simulink model "mdl5"  (R2014a)
settings: Solver=FixedStepDiscrete  SolverMode=SingleTasking  StartTime=TIME(1)  StopTime=TIME(end)  FixedStep=SIMSTEP  RelTol=1e-3
model workspace (MAT data in the model file):
  autoc_mdd_data01 : struct (value not decoded)
values from neighbouring files (symbols this model uses):
  map_mr4_01 = [400 500 600 700 800 900 1000 1100 1200 1300 1400 1500 ... (47 elements, 1x47)]    [scr_simdata_all.mat]
  map_mr4_02 = [0.684 0.622 0.566 0.514 0.468 0.425 0.387 0.352 0.32 0.291 0.264 0.241 ... (47 elements, 1x47)]    [scr_simdata_all.mat]
  map_mr4_03 = [10 12 14 16 18 20 22 24 26 28 30 32 ... (51 elements, 1x51)]    [scr_simdata_all.mat]
  map_mr4_04 = [0.0257 0.0124 0.00595 0.00286 0.00137 0.000662 0.000318 0.000153 7.37e-05 3.54e-05 1.7e-05 8.19e-06 ... (51 elements, 1x51)]    [scr_simdata_all.mat]
  map_mr4_05 = [10 12 14 16 18 20 22 24 26 28 30 32 ... (51 elements, 1x51)]    [scr_simdata_all.mat]
  map_mr4_06 = [0.9647 0.9835 0.9945 0.9994 0.9972 0.9871 0.97 0.9462 0.9163 0.8807 0.8403 0.796 ... (51 elements, 1x51)]    [scr_simdata_all.mat]
  map_mr4_07 = [0 1 2 3 4 5 6 7 8 9 10 11 ... (51 elements, 1x51)]    [scr_simdata_all.mat]
  map_mr4_08 = [0 0.01 0.0214 0.0335 0.0459 0.0587 0.0718 0.085 0.0985 0.112 0.126 0.14 ... (51 elements, 1x51)]    [scr_simdata_all.mat]
  Parameter114 = 126    [scr_simdata_all.mat]
  Parameter115 = 129    [scr_simdata_all.mat]
  Parameter131 = 3    [scr_simdata_all.mat]
  Parameter141 = 0    [scr_simdata_all.mat]
  Parameter143 = 1    [scr_simdata_all.mat]
  Parameter144 = 3    [scr_simdata_all.mat]
  Parameter51 = 0    [scr_simdata_all.mat]
  Parameter52 = 1    [scr_simdata_all.mat]
  Parameter53 = 2    [scr_simdata_all.mat]
  Parameter70 = 30    [scr_simdata_all.mat]
  Parameter71 = 33    [scr_simdata_all.mat]
  Parameter92 = 78    [scr_simdata_all.mat]
  Parameter93 = 81    [scr_simdata_all.mat]
  SIMSTEP = 0.0001024    [scr_simdata_all.mat]
(part 3 of 4)

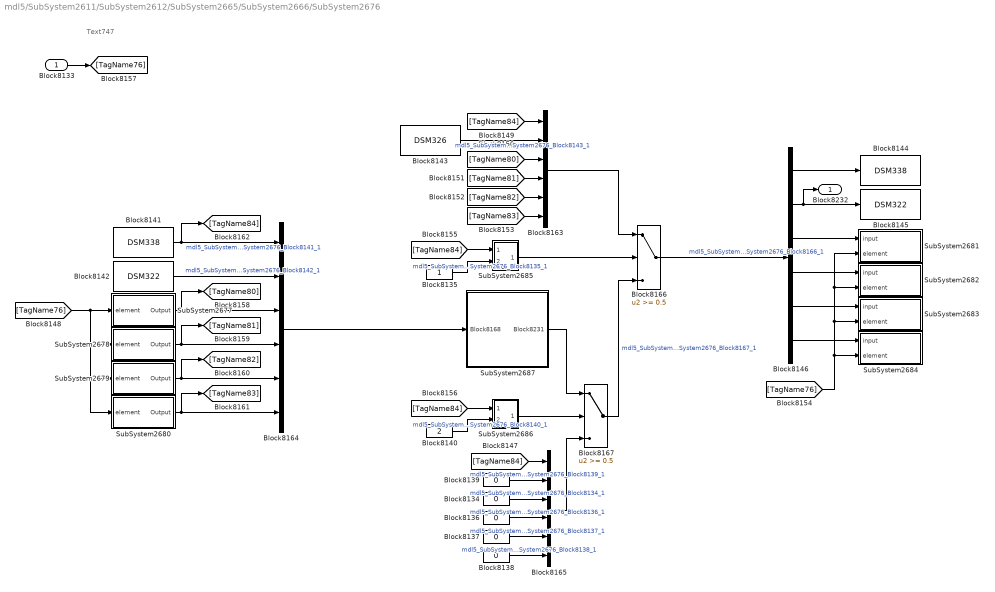
== system mdl5/SubSystem2611/SubSystem2612/SubSystem2665/SubSystem2666/SubSystem2676 ==
  note: Text747
  Block8133 : Inport
  Block{8134,8136..8139} (5 alike) : Constant  Value=0  OutDataTypeStr=double  SampleTime=-1
  Block8135 : Constant  OutDataTypeStr=double  SampleTime=-1
  Block8140 : Constant  Value=2  OutDataTypeStr=double  SampleTime=-1
  Block8141 : DataStoreRead  DataStoreName=DSM338
  Block8142 : DataStoreRead  DataStoreName=DSM322
  Block8143 : DataStoreRead  DataStoreName=DSM326
  Block8144 : DataStoreWrite  DataStoreName=DSM338
  Block8145 : DataStoreWrite  DataStoreName=DSM322
  Block8146 : Demux  Outputs=6
  Block8163 : Mux  Inputs=6
  Block8164 : Mux  Inputs=6
  Block8165 : Mux  Inputs=6
  Block8166 : Switch  Threshold=0.5  RndMeth=Zero  SaturateOnIntegerOverflow=on  InputSameDT=on
  Block8167 : Switch  Threshold=0.5  RndMeth=Zero  SaturateOnIntegerOverflow=on  InputSameDT=on
  SubSystem2677 : Subsystem  TreatAsAtomicUnit=on  mask(***ATC.DSRVEC***){bd_version=1.01.A, r0=DSM334, r1=-1, r2=, r3=, r4=, r5=, r6=, r7=, r8=, r9=, c0=, c1=, c2=, c3=, c4=, c5=, c6=, c7=, c8=, c9=}
      mask prompts: bd_version "Version"
      mask help: これはAutoCからのブロックです．編集禁止．
      settings: OpenFcn=warndlg('変更禁止!');
      mask Help: web(ui_blockhelpmng(gcb));
      mask Display: disp('ATC.DSRVEC')
  SubSystem2678 : Subsystem  TreatAsAtomicUnit=on  mask(***ATC.DSRVEC***){bd_version=1.01.A, r0=DSM335, r1=-1, r2=, r3=, r4=, r5=, r6=, r7=, r8=, r9=, c0=, c1=, c2=, c3=, c4=, c5=, c6=, c7=, c8=, c9=}
      mask prompts: bd_version "Version"
      mask help: これはAutoCからのブロックです．編集禁止．
      settings: OpenFcn=warndlg('変更禁止!');
      mask Help: web(ui_blockhelpmng(gcb));
      mask Display: disp('ATC.DSRVEC')
  SubSystem2679 : Subsystem  TreatAsAtomicUnit=on  mask(***ATC.DSRVEC***){bd_version=1.01.A, r0=DSM336, r1=-1, r2=, r3=, r4=, r5=, r6=, r7=, r8=, r9=, c0=, c1=, c2=, c3=, c4=, c5=, c6=, c7=, c8=, c9=}
      mask prompts: bd_version "Version"
      mask help: これはAutoCからのブロックです．編集禁止．
      settings: OpenFcn=warndlg('変更禁止!');
      mask Help: web(ui_blockhelpmng(gcb));
      mask Display: disp('ATC.DSRVEC')
  SubSystem2680 : Subsystem  TreatAsAtomicUnit=on  mask(***ATC.DSRVEC***){bd_version=1.01.A, r0=DSM337, r1=-1, r2=, r3=, r4=, r5=, r6=, r7=, r8=, r9=, c0=, c1=, c2=, c3=, c4=, c5=, c6=, c7=, c8=, c9=}
      mask prompts: bd_version "Version"
      mask help: これはAutoCからのブロックです．編集禁止．
      settings: OpenFcn=warndlg('変更禁止!');
      mask Help: web(ui_blockhelpmng(gcb));
      mask Display: disp('ATC.DSRVEC')
  SubSystem2681 : Subsystem  TreatAsAtomicUnit=on  mask(***ATC.DSWVEC***){bd_version=1.01.A, r0=DSM334, r1=-1, r2=, r3=, r4=, r5=, r6=, r7=, r8=, r9=, c0=, c1=, c2=, c3=, c4=, c5=, c6=, c7=, c8=, c9=}
      mask prompts: bd_version "Version"
      mask help: これはAutoCからのブロックです．編集禁止．
      settings: OpenFcn=warndlg('変更禁止!');
      mask Help: web(ui_blockhelpmng(gcb));
      mask Display: disp('ATC.DSRVEC')
  SubSystem2682 : Subsystem  TreatAsAtomicUnit=on  mask(***ATC.DSWVEC***){bd_version=1.01.A, r0=DSM335, r1=-1, r2=, r3=, r4=, r5=, r6=, r7=, r8=, r9=, c0=, c1=, c2=, c3=, c4=, c5=, c6=, c7=, c8=, c9=}
      mask prompts: bd_version "Version"
      mask help: これはAutoCからのブロックです．編集禁止．
      settings: OpenFcn=warndlg('変更禁止!');
      mask Help: web(ui_blockhelpmng(gcb));
      mask Display: disp('ATC.DSRVEC')
  SubSystem2683 : Subsystem  TreatAsAtomicUnit=on  mask(***ATC.DSWVEC***){bd_version=1.01.A, r0=DSM336, r1=-1, r2=, r3=, r4=, r5=, r6=, r7=, r8=, r9=, c0=, c1=, c2=, c3=, c4=, c5=, c6=, c7=, c8=, c9=}
      mask prompts: bd_version "Version"
      mask help: これはAutoCからのブロックです．編集禁止．
      settings: OpenFcn=warndlg('変更禁止!');
      mask Help: web(ui_blockhelpmng(gcb));
      mask Display: disp('ATC.DSRVEC')
  SubSystem2684 : Subsystem  TreatAsAtomicUnit=on  mask(***ATC.DSWVEC***){bd_version=1.01.A, r0=DSM337, r1=-1, r2=, r3=, r4=, r5=, r6=, r7=, r8=, r9=, c0=, c1=, c2=, c3=, c4=, c5=, c6=, c7=, c8=, c9=}
      mask prompts: bd_version "Version"
      mask help: これはAutoCからのブロックです．編集禁止．
      settings: OpenFcn=warndlg('変更禁止!');
      mask Help: web(ui_blockhelpmng(gcb));
      mask Display: disp('ATC.DSRVEC')
  SubSystem2685 : Subsystem
  SubSystem2686 : Subsystem
  SubSystem2687 : Subsystem  TreatAsAtomicUnit=on
  Block8232 : Outport
  wires:
  [TagName76] -> SubSystem2681/2(element), SubSystem2682/2(element), SubSystem2683/2(element), SubSystem2684/2(element)
  SubSystem2687/1(Block8231) -> Block8167/1
  Block8133/1 -> [TagName76]
  Block8164/1 -> SubSystem2687/1(Block8168)
  Block8141/1 -> [TagName84], Block8164/1  "mdl5_SubSystem2611_SubSystem2612_SubSystem2665_SubSystem2666_SubSystem2676_Block8141_1"
  Block8142/1 -> Block8164/2  "mdl5_SubSystem2611_SubSystem2612_SubSystem2665_SubSystem2666_SubSystem2676_Block8142_1"
  SubSystem2677/1(Output) -> [TagName80], Block8164/3
  SubSystem2678/1(Output) -> [TagName81], Block8164/4
  SubSystem2679/1(Output) -> [TagName82], Block8164/5
  SubSystem2680/1(Output) -> [TagName83], Block8164/6
  [TagName84] -> SubSystem2685/1(In1)
  Block8135/1 -> SubSystem2685/2(In2)  "mdl5_SubSystem2611_SubSystem2612_SubSystem2665_SubSystem2666_SubSystem2676_Block8135_1"
  [TagName84] -> SubSystem2686/1(In1)
  Block8140/1 -> SubSystem2686/2(In2)  "mdl5_SubSystem2611_SubSystem2612_SubSystem2665_SubSystem2666_SubSystem2676_Block8140_1"
  SubSystem2685/1(Out1) -> Block8166/2
  SubSystem2686/1(Out1) -> Block8167/2
  Block8163/1 -> Block8166/1
  Block8165/1 -> Block8167/3
  [TagName76] -> SubSystem2677/1(element), SubSystem2678/1(element), SubSystem2679/1(element), SubSystem2680/1(element)
  Block8166/1 -> Block8146/1  "mdl5_SubSystem2611_SubSystem2612_SubSystem2665_SubSystem2666_SubSystem2676_Block8166_1"
  Block8167/1 -> Block8166/3  "mdl5_SubSystem2611_SubSystem2612_SubSystem2665_SubSystem2666_SubSystem2676_Block8167_1"
  Block8146/1 -> Block8144/1
  Block8146/2 -> Block8145/1, Block8232/1
  Block8146/3 -> SubSystem2681/1(input)
  Block8146/4 -> SubSystem2682/1(input)
  Block8146/5 -> SubSystem2683/1(input)
  Block8146/6 -> SubSystem2684/1(input)
  [TagName84] -> Block8163/1
  Block8143/1 -> Block8163/2  "mdl5_SubSystem2611_SubSystem2612_SubSystem2665_SubSystem2666_SubSystem2676_Block8143_1"
  [TagName80] -> Block8163/3
  [TagName81] -> Block8163/4
  [TagName82] -> Block8163/5
  [TagName83] -> Block8163/6
  [TagName84] -> Block8165/1
  Block8139/1 -> Block8165/2  "mdl5_SubSystem2611_SubSystem2612_SubSystem2665_SubSystem2666_SubSystem2676_Block8139_1"
  Block8134/1 -> Block8165/3  "mdl5_SubSystem2611_SubSystem2612_SubSystem2665_SubSystem2666_SubSystem2676_Block8134_1"
  Block8136/1 -> Block8165/4  "mdl5_SubSystem2611_SubSystem2612_SubSystem2665_SubSystem2666_SubSystem2676_Block8136_1"
  Block8137/1 -> Block8165/5  "mdl5_SubSystem2611_SubSystem2612_SubSystem2665_SubSystem2666_SubSystem2676_Block8137_1"
  Block8138/1 -> Block8165/6  "mdl5_SubSystem2611_SubSystem2612_SubSystem2665_SubSystem2666_SubSystem2676_Block8138_1"

== system mdl5/SubSystem2611/SubSystem2691/SubSystem2693/SubSystem2695/SubSystem2696 ==
  note: ***編集禁止***
  input : Inport
  element : Inport  Port=2
  Assignment : Assignment  IndexOptions=Index vector (port)  OutputSizes=[1 1]
  Inside_DSR : DataStoreRead  DataStoreName=DSM320
  Inside_DSW : DataStoreWrite  DataStoreName=DSM320
  wires:
  Assignment/1 -> Inside_DSW/1  "mdl5_SubSystem2611_SubSystem2691_SubSystem2693_SubSystem2695_SubSystem2696_Assignment_1"
  Inside_DSR/1 -> Assignment/1  "mdl5_SubSystem2611_SubSystem2691_SubSystem2693_SubSystem2695_SubSystem2696_Inside_DSR_1"
  input/1 -> Assignment/2
  element/1 -> Assignment/3

== system mdl5/SubSystem2611/SubSystem2691/SubSystem2693/SubSystem2695/SubSystem2697 ==
  note: ***編集禁止***
  input : Inport
  element : Inport  Port=2
  Assignment : Assignment  IndexOptions=Index vector (port)  OutputSizes=[1 1]
  Inside_DSR : DataStoreRead  DataStoreName=DSM319
  Inside_DSW : DataStoreWrite  DataStoreName=DSM319
  wires:
  Assignment/1 -> Inside_DSW/1  "mdl5_SubSystem2611_SubSystem2691_SubSystem2693_SubSystem2695_SubSystem2697_Assignment_1"
  Inside_DSR/1 -> Assignment/1  "mdl5_SubSystem2611_SubSystem2691_SubSystem2693_SubSystem2695_SubSystem2697_Inside_DSR_1"
  input/1 -> Assignment/2
  element/1 -> Assignment/3

== system mdl5/SubSystem2611/SubSystem2691/SubSystem2693/SubSystem2695/SubSystem2698 ==
  note: ***編集禁止***
  input : Inport
  element : Inport  Port=2
  Assignment : Assignment  IndexOptions=Index vector (port)  OutputSizes=[1 1]
  Inside_DSR : DataStoreRead  DataStoreName=DSM336
  Inside_DSW : DataStoreWrite  DataStoreName=DSM336
  wires:
  element/1 -> Assignment/3
  input/1 -> Assignment/2
  Inside_DSR/1 -> Assignment/1  "mdl5_SubSystem2611_SubSystem2691_SubSystem2693_SubSystem2695_SubSystem2698_Inside_DSR_1"
  Assignment/1 -> Inside_DSW/1  "mdl5_SubSystem2611_SubSystem2691_SubSystem2693_SubSystem2695_SubSystem2698_Assignment_1"

== system mdl5/SubSystem2611/SubSystem2691/SubSystem2693/SubSystem2695/SubSystem2699 ==
  note: ***編集禁止***
  input : Inport
  element : Inport  Port=2
  Assignment : Assignment  IndexOptions=Index vector (port)  OutputSizes=[1 1]
  Inside_DSR : DataStoreRead  DataStoreName=DSM318
  Inside_DSW : DataStoreWrite  DataStoreName=DSM318
  wires:
  Assignment/1 -> Inside_DSW/1  "mdl5_SubSystem2611_SubSystem2691_SubSystem2693_SubSystem2695_SubSystem2699_Assignment_1"
  Inside_DSR/1 -> Assignment/1  "mdl5_SubSystem2611_SubSystem2691_SubSystem2693_SubSystem2695_SubSystem2699_Inside_DSR_1"
  input/1 -> Assignment/2
  element/1 -> Assignment/3

== system mdl5/SubSystem2611/SubSystem2691/SubSystem2693/SubSystem2695/SubSystem2700 ==
  note: ***編集禁止***
  input : Inport
  element : Inport  Port=2
  Assignment : Assignment  IndexOptions=Index vector (port)  OutputSizes=[1 1]
  Inside_DSR : DataStoreRead  DataStoreName=DSM333
  Inside_DSW : DataStoreWrite  DataStoreName=DSM333
  wires:
  element/1 -> Assignment/3
  input/1 -> Assignment/2
  Inside_DSR/1 -> Assignment/1  "mdl5_SubSystem2611_SubSystem2691_SubSystem2693_SubSystem2695_SubSystem2700_Inside_DSR_1"
  Assignment/1 -> Inside_DSW/1  "mdl5_SubSystem2611_SubSystem2691_SubSystem2693_SubSystem2695_SubSystem2700_Assignment_1"

== system mdl5/SubSystem2611/SubSystem2691/SubSystem2693/SubSystem2695/SubSystem2701 ==
  note: ***編集禁止***
  input : Inport
  element : Inport  Port=2
  Assignment : Assignment  IndexOptions=Index vector (port)  OutputSizes=[1 1]
  Inside_DSR : DataStoreRead  DataStoreName=DSM337
  Inside_DSW : DataStoreWrite  DataStoreName=DSM337
  wires:
  Assignment/1 -> Inside_DSW/1  "mdl5_SubSystem2611_SubSystem2691_SubSystem2693_SubSystem2695_SubSystem2701_Assignment_1"
  Inside_DSR/1 -> Assignment/1  "mdl5_SubSystem2611_SubSystem2691_SubSystem2693_SubSystem2695_SubSystem2701_Inside_DSR_1"
  input/1 -> Assignment/2
  element/1 -> Assignment/3

== system mdl5/SubSystem2611/SubSystem2691/SubSystem2693/SubSystem2695/SubSystem2702 ==
  note: ***編集禁止***
  input : Inport
  element : Inport  Port=2
  Assignment : Assignment  IndexOptions=Index vector (port)  OutputSizes=[1 1]
  Inside_DSR : DataStoreRead  DataStoreName=DSM334
  Inside_DSW : DataStoreWrite  DataStoreName=DSM334
  wires:
  element/1 -> Assignment/3
  input/1 -> Assignment/2
  Inside_DSR/1 -> Assignment/1  "mdl5_SubSystem2611_SubSystem2691_SubSystem2693_SubSystem2695_SubSystem2702_Inside_DSR_1"
  Assignment/1 -> Inside_DSW/1  "mdl5_SubSystem2611_SubSystem2691_SubSystem2693_SubSystem2695_SubSystem2702_Assignment_1"

== system mdl5/SubSystem2611/SubSystem2691/SubSystem2693/SubSystem2695/SubSystem2703 ==
  note: ***編集禁止***
  input : Inport
  element : Inport  Port=2
  Assignment : Assignment  IndexOptions=Index vector (port)  OutputSizes=[1 1]
  Inside_DSR : DataStoreRead  DataStoreName=DSM335
  Inside_DSW : DataStoreWrite  DataStoreName=DSM335
  wires:
  element/1 -> Assignment/3
  input/1 -> Assignment/2
  Inside_DSR/1 -> Assignment/1  "mdl5_SubSystem2611_SubSystem2691_SubSystem2693_SubSystem2695_SubSystem2703_Inside_DSR_1"
  Assignment/1 -> Inside_DSW/1  "mdl5_SubSystem2611_SubSystem2691_SubSystem2693_SubSystem2695_SubSystem2703_Assignment_1"

== system mdl5/SubSystem2611/SubSystem2691/SubSystem2693/SubSystem2695/SubSystem2704 ==
  note: ***編集禁止***
  input : Inport
  element : Inport  Port=2
  Assignment : Assignment  IndexOptions=Index vector (port)  OutputSizes=[1 1]
  Inside_DSR : DataStoreRead  DataStoreName=DSM348
  Inside_DSW : DataStoreWrite  DataStoreName=DSM348
  wires:
  Assignment/1 -> Inside_DSW/1  "mdl5_SubSystem2611_SubSystem2691_SubSystem2693_SubSystem2695_SubSystem2704_Assignment_1"
  Inside_DSR/1 -> Assignment/1  "mdl5_SubSystem2611_SubSystem2691_SubSystem2693_SubSystem2695_SubSystem2704_Inside_DSR_1"
  input/1 -> Assignment/2
  element/1 -> Assignment/3

== system mdl5/SubSystem2611/SubSystem2691/SubSystem2693/SubSystem2695/SubSystem2705 ==
  note: ***編集禁止***
  input : Inport
  element : Inport  Port=2
  Assignment : Assignment  IndexOptions=Index vector (port)  OutputSizes=[1 1]
  Inside_DSR : DataStoreRead  DataStoreName=DSM349
  Inside_DSW : DataStoreWrite  DataStoreName=DSM349
  wires:
  Assignment/1 -> Inside_DSW/1  "mdl5_SubSystem2611_SubSystem2691_SubSystem2693_SubSystem2695_SubSystem2705_Assignment_1"
  Inside_DSR/1 -> Assignment/1  "mdl5_SubSystem2611_SubSystem2691_SubSystem2693_SubSystem2695_SubSystem2705_Inside_DSR_1"
  input/1 -> Assignment/2
  element/1 -> Assignment/3

== system mdl5/SubSystem2611/SubSystem2691/SubSystem2693/SubSystem2695/SubSystem2706 ==
  note: ***編集禁止***
  input : Inport
  element : Inport  Port=2
  Assignment : Assignment  IndexOptions=Index vector (port)  OutputSizes=[1 1]
  Inside_DSR : DataStoreRead  DataStoreName=DSM347
  Inside_DSW : DataStoreWrite  DataStoreName=DSM347
  wires:
  Assignment/1 -> Inside_DSW/1  "mdl5_SubSystem2611_SubSystem2691_SubSystem2693_SubSystem2695_SubSystem2706_Assignment_1"
  Inside_DSR/1 -> Assignment/1  "mdl5_SubSystem2611_SubSystem2691_SubSystem2693_SubSystem2695_SubSystem2706_Inside_DSR_1"
  input/1 -> Assignment/2
  element/1 -> Assignment/3

== system mdl5/SubSystem2611/SubSystem2612/SubSystem2620/SubSystem2624/SubSystem2627/SubSystem2628 ==
  note: ***編集禁止***
  element : Inport
  Inside_DSR : DataStoreRead  DataStoreName=DSM147
  Selector : Selector  IndexOptions=Index vector (port)  Indices=[1 3]
  Output : Outport
  wires:
  Selector/1 -> Output/1  "mdl5_SubSystem2611_SubSystem2612_SubSystem2620_SubSystem2624_SubSystem2627_SubSystem2628_Selector_1"
  element/1 -> Selector/2
  Inside_DSR/1 -> Selector/1  "mdl5_SubSystem2611_SubSystem2612_SubSystem2620_SubSystem2624_SubSystem2627_SubSystem2628_Inside_DSR_1"

== system mdl5/SubSystem2611/SubSystem2612/SubSystem2620/SubSystem2624/SubSystem2627/SubSystem2629 ==
  note: ***編集禁止***
  element : Inport
  Inside_DSR : DataStoreRead  DataStoreName=DSM304
  Selector : Selector  IndexOptions=Index vector (port)  Indices=[1 3]
  Output : Outport
  wires:
  Inside_DSR/1 -> Selector/1  "mdl5_SubSystem2611_SubSystem2612_SubSystem2620_SubSystem2624_SubSystem2627_SubSystem2629_Inside_DSR_1"
  element/1 -> Selector/2
  Selector/1 -> Output/1  "mdl5_SubSystem2611_SubSystem2612_SubSystem2620_SubSystem2624_SubSystem2627_SubSystem2629_Selector_1"

== system mdl5/SubSystem2611/SubSystem2612/SubSystem2620/SubSystem2624/SubSystem2627/SubSystem2630 ==
  note: ***編集禁止***
  element : Inport
  Inside_DSR : DataStoreRead  DataStoreName=DSM346
  Selector : Selector  IndexOptions=Index vector (port)  Indices=[1 3]
  Output : Outport
  wires:
  Selector/1 -> Output/1  "mdl5_SubSystem2611_SubSystem2612_SubSystem2620_SubSystem2624_SubSystem2627_SubSystem2630_Selector_1"
  element/1 -> Selector/2
  Inside_DSR/1 -> Selector/1  "mdl5_SubSystem2611_SubSystem2612_SubSystem2620_SubSystem2624_SubSystem2627_SubSystem2630_Inside_DSR_1"

== system mdl5/SubSystem2611/SubSystem2612/SubSystem2620/SubSystem2624/SubSystem2627/SubSystem2631 ==
  note: ***編集禁止***
  input : Inport
  element : Inport  Port=2
  Assignment : Assignment  IndexOptions=Index vector (port)  OutputSizes=[1 1]
  Inside_DSR : DataStoreRead  DataStoreName=DSM346
  Inside_DSW : DataStoreWrite  DataStoreName=DSM346
  wires:
  Assignment/1 -> Inside_DSW/1  "mdl5_SubSystem2611_SubSystem2612_SubSystem2620_SubSystem2624_SubSystem2627_SubSystem2631_Assignment_1"
  Inside_DSR/1 -> Assignment/1  "mdl5_SubSystem2611_SubSystem2612_SubSystem2620_SubSystem2624_SubSystem2627_SubSystem2631_Inside_DSR_1"
  input/1 -> Assignment/2
  element/1 -> Assignment/3

== system mdl5/SubSystem2611/SubSystem2612/SubSystem2620/SubSystem2624/SubSystem2627/SubSystem2632 ==
  note: ***編集禁止***
  input : Inport
  element : Inport  Port=2
  Assignment : Assignment  IndexOptions=Index vector (port)  OutputSizes=[1 1]
  Inside_DSR : DataStoreRead  DataStoreName=DSM349
  Inside_DSW : DataStoreWrite  DataStoreName=DSM349
  wires:
  Assignment/1 -> Inside_DSW/1  "mdl5_SubSystem2611_SubSystem2612_SubSystem2620_SubSystem2624_SubSystem2627_SubSystem2632_Assignment_1"
  Inside_DSR/1 -> Assignment/1  "mdl5_SubSystem2611_SubSystem2612_SubSystem2620_SubSystem2624_SubSystem2627_SubSystem2632_Inside_DSR_1"
  input/1 -> Assignment/2
  element/1 -> Assignment/3

== system mdl5/SubSystem2611/SubSystem2612/SubSystem2620/SubSystem2624/SubSystem2627/SubSystem2633 ==
  note: ***編集禁止***
  input : Inport
  element : Inport  Port=2
  Assignment : Assignment  IndexOptions=Index vector (port)  OutputSizes=[1 1]
  Inside_DSR : DataStoreRead  DataStoreName=DSM348
  Inside_DSW : DataStoreWrite  DataStoreName=DSM348
  wires:
  element/1 -> Assignment/3
  input/1 -> Assignment/2
  Inside_DSR/1 -> Assignment/1  "mdl5_SubSystem2611_SubSystem2612_SubSystem2620_SubSystem2624_SubSystem2627_SubSystem2633_Inside_DSR_1"
  Assignment/1 -> Inside_DSW/1  "mdl5_SubSystem2611_SubSystem2612_SubSystem2620_SubSystem2624_SubSystem2627_SubSystem2633_Assignment_1"

== system mdl5/SubSystem2611/SubSystem2612/SubSystem2620/SubSystem2624/SubSystem2627/SubSystem2634 ==
  note: ***編集禁止***
  input : Inport
  element : Inport  Port=2
  Assignment : Assignment  IndexOptions=Index vector (port)  OutputSizes=[1 1]
  Inside_DSR : DataStoreRead  DataStoreName=DSM347
  Inside_DSW : DataStoreWrite  DataStoreName=DSM347
  wires:
  element/1 -> Assignment/3
  input/1 -> Assignment/2
  Inside_DSR/1 -> Assignment/1  "mdl5_SubSystem2611_SubSystem2612_SubSystem2620_SubSystem2624_SubSystem2627_SubSystem2634_Inside_DSR_1"
  Assignment/1 -> Inside_DSW/1  "mdl5_SubSystem2611_SubSystem2612_SubSystem2620_SubSystem2624_SubSystem2627_SubSystem2634_Assignment_1"

== system mdl5/SubSystem2611/SubSystem2612/SubSystem2620/SubSystem2624/SubSystem2627/SubSystem2635 ==
  note: ***編集禁止***
  In1 : Inport
  In2 : Inport  Port=2
  RO1 : RelationalOperator  Operator===  InputSameDT=on
  single1 : DataTypeConversion  OutDataTypeStr=single  SaturateOnIntegerOverflow=on  RndMeth=Zero
  single2 : DataTypeConversion  OutDataTypeStr=single  SaturateOnIntegerOverflow=on  RndMeth=Zero
  Out1 : Outport
  wires:
  single2/1 -> RO1/2  "mdl5_SubSystem2611_SubSystem2612_SubSystem2620_SubSystem2624_SubSystem2627_SubSystem2635_single2_1"
  single1/1 -> RO1/1  "mdl5_SubSystem2611_SubSystem2612_SubSystem2620_SubSystem2624_SubSystem2627_SubSystem2635_single1_1"
  In1/1 -> single1/1
  In2/1 -> single2/1
  RO1/1 -> Out1/1  "mdl5_SubSystem2611_SubSystem2612_SubSystem2620_SubSystem2624_SubSystem2627_SubSystem2635_RO1_1"

== system mdl5/SubSystem2611/SubSystem2612/SubSystem2620/SubSystem2624/SubSystem2638/SubSystem2639 ==
  note: ***編集禁止***
  element : Inport
  Inside_DSR : DataStoreRead  DataStoreName=DSM97
  Selector : Selector  IndexOptions=Index vector (port)  Indices=[1 3]
  Output : Outport
  wires:
  Inside_DSR/1 -> Selector/1  "mdl5_SubSystem2611_SubSystem2612_SubSystem2620_SubSystem2624_SubSystem2638_SubSystem2639_Inside_DSR_1"
  element/1 -> Selector/2
  Selector/1 -> Output/1  "mdl5_SubSystem2611_SubSystem2612_SubSystem2620_SubSystem2624_SubSystem2638_SubSystem2639_Selector_1"

== system mdl5/SubSystem2611/SubSystem2612/SubSystem2620/SubSystem2624/SubSystem2638/SubSystem2640 ==
  note: ***編集禁止***
  element : Inport
  Inside_DSR : DataStoreRead  DataStoreName=DSM318
  Selector : Selector  IndexOptions=Index vector (port)  Indices=[1 3]
  Output : Outport
  wires:
  Selector/1 -> Output/1  "mdl5_SubSystem2611_SubSystem2612_SubSystem2620_SubSystem2624_SubSystem2638_SubSystem2640_Selector_1"
  element/1 -> Selector/2
  Inside_DSR/1 -> Selector/1  "mdl5_SubSystem2611_SubSystem2612_SubSystem2620_SubSystem2624_SubSystem2638_SubSystem2640_Inside_DSR_1"

== system mdl5/SubSystem2611/SubSystem2612/SubSystem2620/SubSystem2624/SubSystem2638/SubSystem2641 ==
  note: ***編集禁止***
  mult : Inport
  div : Inport  Port=2
  Product : Product  Inputs=*/  SaturateOnIntegerOverflow=on  RndMeth=Zero  InputSameDT=on  OutDataTypeStr=Inherit: Same as first input
  Out : Outport
  wires:
  div/1 -> Product/2
  mult/1 -> Product/1
  Product/1 -> Out/1

== system mdl5/SubSystem2611/SubSystem2612/SubSystem2620/SubSystem2624/SubSystem2638/SubSystem2642 ==
  note: ***編集禁止***
  mult : Inport
  div : Inport  Port=2
  Product : Product  Inputs=*/  SaturateOnIntegerOverflow=on  RndMeth=Zero  InputSameDT=on  OutDataTypeStr=Inherit: Same as first input
  Out : Outport
  wires:
  Product/1 -> Out/1  "mdl5_SubSystem2611_SubSystem2612_SubSystem2620_SubSystem2624_SubSystem2638_SubSystem2642_Product_1"
  mult/1 -> Product/1
  div/1 -> Product/2

== system mdl5/SubSystem2611/SubSystem2612/SubSystem2620/SubSystem2624/SubSystem2638/SubSystem2643 ==
  note: ***編集禁止***
  Max : Inport
  Input : Inport  Port=2
  Min1 : MinMax  Inputs=2  SaturateOnIntegerOverflow=on  InputSameDT=on
  Output : Outport
  wires:
  Max/1 -> Min1/1
  Input/1 -> Min1/2
  Min1/1 -> Output/1  "mdl5_SubSystem2611_SubSystem2612_SubSystem2620_SubSystem2624_SubSystem2638_SubSystem2643_Min1_1"

== system mdl5/SubSystem2611/SubSystem2612/SubSystem2620/SubSystem2624/SubSystem2644/SubSystem2645 ==
  note: ***編集禁止***
  element : Inport
  Inside_DSR : DataStoreRead  DataStoreName=DSM115
  Selector : Selector  IndexOptions=Index vector (port)  Indices=[1 3]
  Output : Outport
  wires:
  Inside_DSR/1 -> Selector/1  "mdl5_SubSystem2611_SubSystem2612_SubSystem2620_SubSystem2624_SubSystem2644_SubSystem2645_Inside_DSR_1"
  element/1 -> Selector/2
  Selector/1 -> Output/1  "mdl5_SubSystem2611_SubSystem2612_SubSystem2620_SubSystem2624_SubSystem2644_SubSystem2645_Selector_1"

== system mdl5/SubSystem2611/SubSystem2612/SubSystem2620/SubSystem2624/SubSystem2644/SubSystem2646 ==
  note: ***編集禁止***
  element : Inport
  Inside_DSR : DataStoreRead  DataStoreName=DSM119
  Selector : Selector  IndexOptions=Index vector (port)  Indices=[1 3]
  Output : Outport
  wires:
  Selector/1 -> Output/1  "mdl5_SubSystem2611_SubSystem2612_SubSystem2620_SubSystem2624_SubSystem2644_SubSystem2646_Selector_1"
  element/1 -> Selector/2
  Inside_DSR/1 -> Selector/1  "mdl5_SubSystem2611_SubSystem2612_SubSystem2620_SubSystem2624_SubSystem2644_SubSystem2646_Inside_DSR_1"

== system mdl5/SubSystem2611/SubSystem2612/SubSystem2620/SubSystem2624/SubSystem2644/SubSystem2647 ==
  note: ***編集禁止***
  element : Inport
  Inside_DSR : DataStoreRead  DataStoreName=DSM102
  Selector : Selector  IndexOptions=Index vector (port)  Indices=[1 3]
  Output : Outport
  wires:
  Selector/1 -> Output/1  "mdl5_SubSystem2611_SubSystem2612_SubSystem2620_SubSystem2624_SubSystem2644_SubSystem2647_Selector_1"
  element/1 -> Selector/2
  Inside_DSR/1 -> Selector/1  "mdl5_SubSystem2611_SubSystem2612_SubSystem2620_SubSystem2624_SubSystem2644_SubSystem2647_Inside_DSR_1"

== system mdl5/SubSystem2611/SubSystem2612/SubSystem2620/SubSystem2624/SubSystem2644/SubSystem2648 ==
  note: ***編集禁止***
  element : Inport
  Inside_DSR : DataStoreRead  DataStoreName=DSM104
  Selector : Selector  IndexOptions=Index vector (port)  Indices=[1 3]
  Output : Outport
  wires:
  Inside_DSR/1 -> Selector/1  "mdl5_SubSystem2611_SubSystem2612_SubSystem2620_SubSystem2624_SubSystem2644_SubSystem2648_Inside_DSR_1"
  element/1 -> Selector/2
  Selector/1 -> Output/1  "mdl5_SubSystem2611_SubSystem2612_SubSystem2620_SubSystem2624_SubSystem2644_SubSystem2648_Selector_1"

== system mdl5/SubSystem2611/SubSystem2612/SubSystem2620/SubSystem2624/SubSystem2644/SubSystem2649 ==
  note: ***編集禁止***
  element : Inport
  Inside_DSR : DataStoreRead  DataStoreName=DSM110
  Selector : Selector  IndexOptions=Index vector (port)  Indices=[1 3]
  Output : Outport
  wires:
  Inside_DSR/1 -> Selector/1  "mdl5_SubSystem2611_SubSystem2612_SubSystem2620_SubSystem2624_SubSystem2644_SubSystem2649_Inside_DSR_1"
  element/1 -> Selector/2
  Selector/1 -> Output/1  "mdl5_SubSystem2611_SubSystem2612_SubSystem2620_SubSystem2624_SubSystem2644_SubSystem2649_Selector_1"

== system mdl5/SubSystem2611/SubSystem2612/SubSystem2620/SubSystem2624/SubSystem2644/SubSystem2650 ==
  note: ***編集禁止***
  element : Inport
  Inside_DSR : DataStoreRead  DataStoreName=DSM112
  Selector : Selector  IndexOptions=Index vector (port)  Indices=[1 3]
  Output : Outport
  wires:
  Selector/1 -> Output/1  "mdl5_SubSystem2611_SubSystem2612_SubSystem2620_SubSystem2624_SubSystem2644_SubSystem2650_Selector_1"
  element/1 -> Selector/2
  Inside_DSR/1 -> Selector/1  "mdl5_SubSystem2611_SubSystem2612_SubSystem2620_SubSystem2624_SubSystem2644_SubSystem2650_Inside_DSR_1"

== system mdl5/SubSystem2611/SubSystem2612/SubSystem2620/SubSystem2624/SubSystem2644/SubSystem2651 ==
  note: ***編集禁止***
  element : Inport
  Inside_DSR : DataStoreRead  DataStoreName=DSM116
  Selector : Selector  IndexOptions=Index vector (port)  Indices=[1 3]
  Output : Outport
  wires:
  Selector/1 -> Output/1  "mdl5_SubSystem2611_SubSystem2612_SubSystem2620_SubSystem2624_SubSystem2644_SubSystem2651_Selector_1"
  element/1 -> Selector/2
  Inside_DSR/1 -> Selector/1  "mdl5_SubSystem2611_SubSystem2612_SubSystem2620_SubSystem2624_SubSystem2644_SubSystem2651_Inside_DSR_1"

== system mdl5/SubSystem2611/SubSystem2612/SubSystem2620/SubSystem2624/SubSystem2644/SubSystem2652 ==
  note: ***編集禁止***
  element : Inport
  Inside_DSR : DataStoreRead  DataStoreName=DSM120
  Selector : Selector  IndexOptions=Index vector (port)  Indices=[1 3]
  Output : Outport
  wires:
  Inside_DSR/1 -> Selector/1  "mdl5_SubSystem2611_SubSystem2612_SubSystem2620_SubSystem2624_SubSystem2644_SubSystem2652_Inside_DSR_1"
  element/1 -> Selector/2
  Selector/1 -> Output/1  "mdl5_SubSystem2611_SubSystem2612_SubSystem2620_SubSystem2624_SubSystem2644_SubSystem2652_Selector_1"

== system mdl5/SubSystem2611/SubSystem2612/SubSystem2620/SubSystem2624/SubSystem2644/SubSystem2653 ==
  note: ***編集禁止***
  element : Inport
  Inside_DSR : DataStoreRead  DataStoreName=DSM122
  Selector : Selector  IndexOptions=Index vector (port)  Indices=[1 3]
  Output : Outport
  wires:
  Inside_DSR/1 -> Selector/1  "mdl5_SubSystem2611_SubSystem2612_SubSystem2620_SubSystem2624_SubSystem2644_SubSystem2653_Inside_DSR_1"
  element/1 -> Selector/2
  Selector/1 -> Output/1  "mdl5_SubSystem2611_SubSystem2612_SubSystem2620_SubSystem2624_SubSystem2644_SubSystem2653_Selector_1"

== system mdl5/SubSystem2611/SubSystem2612/SubSystem2620/SubSystem2624/SubSystem2644/SubSystem2654 ==
  note: ***編集禁止***
  element : Inport
  Inside_DSR : DataStoreRead  DataStoreName=DSM125
  Selector : Selector  IndexOptions=Index vector (port)  Indices=[1 3]
  Output : Outport
  wires:
  Selector/1 -> Output/1  "mdl5_SubSystem2611_SubSystem2612_SubSystem2620_SubSystem2624_SubSystem2644_SubSystem2654_Selector_1"
  element/1 -> Selector/2
  Inside_DSR/1 -> Selector/1  "mdl5_SubSystem2611_SubSystem2612_SubSystem2620_SubSystem2624_SubSystem2644_SubSystem2654_Inside_DSR_1"

== system mdl5/SubSystem2611/SubSystem2612/SubSystem2620/SubSystem2624/SubSystem2644/SubSystem2655 ==
  note: ***編集禁止***
  element : Inport
  Inside_DSR : DataStoreRead  DataStoreName=DSM123
  Selector : Selector  IndexOptions=Index vector (port)  Indices=[1 3]
  Output : Outport
  wires:
  Selector/1 -> Output/1  "mdl5_SubSystem2611_SubSystem2612_SubSystem2620_SubSystem2624_SubSystem2644_SubSystem2655_Selector_1"
  element/1 -> Selector/2
  Inside_DSR/1 -> Selector/1  "mdl5_SubSystem2611_SubSystem2612_SubSystem2620_SubSystem2624_SubSystem2644_SubSystem2655_Inside_DSR_1"

== system mdl5/SubSystem2611/SubSystem2612/SubSystem2620/SubSystem2624/SubSystem2644/SubSystem2656 ==
  note: ***編集禁止***
  element : Inport
  Inside_DSR : DataStoreRead  DataStoreName=DSM126
  Selector : Selector  IndexOptions=Index vector (port)  Indices=[1 3]
  Output : Outport
  wires:
  Inside_DSR/1 -> Selector/1  "mdl5_SubSystem2611_SubSystem2612_SubSystem2620_SubSystem2624_SubSystem2644_SubSystem2656_Inside_DSR_1"
  element/1 -> Selector/2
  Selector/1 -> Output/1  "mdl5_SubSystem2611_SubSystem2612_SubSystem2620_SubSystem2624_SubSystem2644_SubSystem2656_Selector_1"

== system mdl5/SubSystem2611/SubSystem2612/SubSystem2620/SubSystem2624/SubSystem2644/SubSystem2657 ==
  note: ***編集禁止***
  element : Inport
  Inside_DSR : DataStoreRead  DataStoreName=DSM106
  Selector : Selector  IndexOptions=Index vector (port)  Indices=[1 3]
  Output : Outport
  wires:
  Inside_DSR/1 -> Selector/1  "mdl5_SubSystem2611_SubSystem2612_SubSystem2620_SubSystem2624_SubSystem2644_SubSystem2657_Inside_DSR_1"
  element/1 -> Selector/2
  Selector/1 -> Output/1  "mdl5_SubSystem2611_SubSystem2612_SubSystem2620_SubSystem2624_SubSystem2644_SubSystem2657_Selector_1"

== system mdl5/SubSystem2611/SubSystem2612/SubSystem2620/SubSystem2624/SubSystem2644/SubSystem2658 ==
  note: ***編集禁止***
  element : Inport
  Inside_DSR : DataStoreRead  DataStoreName=DSM108
  Selector : Selector  IndexOptions=Index vector (port)  Indices=[1 3]
  Output : Outport
  wires:
  Selector/1 -> Output/1  "mdl5_SubSystem2611_SubSystem2612_SubSystem2620_SubSystem2624_SubSystem2644_SubSystem2658_Selector_1"
  element/1 -> Selector/2
  Inside_DSR/1 -> Selector/1  "mdl5_SubSystem2611_SubSystem2612_SubSystem2620_SubSystem2624_SubSystem2644_SubSystem2658_Inside_DSR_1"

== system mdl5/SubSystem2611/SubSystem2612/SubSystem2620/SubSystem2624/SubSystem2644/SubSystem2659 ==
  note: ***編集禁止***
  In1 : Inport
  In2 : Inport  Port=2
  RO1 : RelationalOperator  Operator===  InputSameDT=on
  single1 : DataTypeConversion  OutDataTypeStr=single  SaturateOnIntegerOverflow=on  RndMeth=Zero
  single2 : DataTypeConversion  OutDataTypeStr=single  SaturateOnIntegerOverflow=on  RndMeth=Zero
  Out1 : Outport
  wires:
  single2/1 -> RO1/2  "mdl5_SubSystem2611_SubSystem2612_SubSystem2620_SubSystem2624_SubSystem2644_SubSystem2659_single2_1"
  single1/1 -> RO1/1  "mdl5_SubSystem2611_SubSystem2612_SubSystem2620_SubSystem2624_SubSystem2644_SubSystem2659_single1_1"
  In1/1 -> single1/1
  In2/1 -> single2/1
  RO1/1 -> Out1/1  "mdl5_SubSystem2611_SubSystem2612_SubSystem2620_SubSystem2624_SubSystem2644_SubSystem2659_RO1_1"

== system mdl5/SubSystem2611/SubSystem2612/SubSystem2620/SubSystem2624/SubSystem2644/SubSystem2660 ==
  note: ***編集禁止***
  In1 : Inport
  In2 : Inport  Port=2
  RO1 : RelationalOperator  Operator===  InputSameDT=on
  single1 : DataTypeConversion  OutDataTypeStr=single  SaturateOnIntegerOverflow=on  RndMeth=Zero
  single2 : DataTypeConversion  OutDataTypeStr=single  SaturateOnIntegerOverflow=on  RndMeth=Zero
  Out1 : Outport
  wires:
  RO1/1 -> Out1/1  "mdl5_SubSystem2611_SubSystem2612_SubSystem2620_SubSystem2624_SubSystem2644_SubSystem2660_RO1_1"
  In2/1 -> single2/1
  In1/1 -> single1/1
  single1/1 -> RO1/1  "mdl5_SubSystem2611_SubSystem2612_SubSystem2620_SubSystem2624_SubSystem2644_SubSystem2660_single1_1"
  single2/1 -> RO1/2  "mdl5_SubSystem2611_SubSystem2612_SubSystem2620_SubSystem2624_SubSystem2644_SubSystem2660_single2_1"

== system mdl5/SubSystem2611/SubSystem2612/SubSystem2620/SubSystem2624/SubSystem2644/SubSystem2661 ==
  note: ***編集禁止***
  In1 : Inport
  In2 : Inport  Port=2
  RO1 : RelationalOperator  Operator===  InputSameDT=on
  single1 : DataTypeConversion  OutDataTypeStr=single  SaturateOnIntegerOverflow=on  RndMeth=Zero
  single2 : DataTypeConversion  OutDataTypeStr=single  SaturateOnIntegerOverflow=on  RndMeth=Zero
  Out1 : Outport
  wires:
  single2/1 -> RO1/2  "mdl5_SubSystem2611_SubSystem2612_SubSystem2620_SubSystem2624_SubSystem2644_SubSystem2661_single2_1"
  single1/1 -> RO1/1  "mdl5_SubSystem2611_SubSystem2612_SubSystem2620_SubSystem2624_SubSystem2644_SubSystem2661_single1_1"
  In1/1 -> single1/1
  In2/1 -> single2/1
  RO1/1 -> Out1/1  "mdl5_SubSystem2611_SubSystem2612_SubSystem2620_SubSystem2624_SubSystem2644_SubSystem2661_RO1_1"

== system mdl5/SubSystem2611/SubSystem2612/SubSystem2620/SubSystem2624/SubSystem2644/SubSystem2662 ==
  note: ***編集禁止***
  In1 : Inport
  In2 : Inport  Port=2
  RO1 : RelationalOperator  Operator===  InputSameDT=on
  single1 : DataTypeConversion  OutDataTypeStr=single  SaturateOnIntegerOverflow=on  RndMeth=Zero
  single2 : DataTypeConversion  OutDataTypeStr=single  SaturateOnIntegerOverflow=on  RndMeth=Zero
  Out1 : Outport
  wires:
  RO1/1 -> Out1/1  "mdl5_SubSystem2611_SubSystem2612_SubSystem2620_SubSystem2624_SubSystem2644_SubSystem2662_RO1_1"
  In2/1 -> single2/1
  In1/1 -> single1/1
  single1/1 -> RO1/1  "mdl5_SubSystem2611_SubSystem2612_SubSystem2620_SubSystem2624_SubSystem2644_SubSystem2662_single1_1"
  single2/1 -> RO1/2  "mdl5_SubSystem2611_SubSystem2612_SubSystem2620_SubSystem2624_SubSystem2644_SubSystem2662_single2_1"

== system mdl5/SubSystem2611/SubSystem2612/SubSystem2620/SubSystem2624/SubSystem2644/SubSystem2663 ==
  note: ***編集禁止***
  In1 : Inport
  In2 : Inport  Port=2
  RO1 : RelationalOperator  Operator===  InputSameDT=on
  single1 : DataTypeConversion  OutDataTypeStr=single  SaturateOnIntegerOverflow=on  RndMeth=Zero
  single2 : DataTypeConversion  OutDataTypeStr=single  SaturateOnIntegerOverflow=on  RndMeth=Zero
  Out1 : Outport
  wires:
  RO1/1 -> Out1/1  "mdl5_SubSystem2611_SubSystem2612_SubSystem2620_SubSystem2624_SubSystem2644_SubSystem2663_RO1_1"
  In2/1 -> single2/1
  In1/1 -> single1/1
  single1/1 -> RO1/1  "mdl5_SubSystem2611_SubSystem2612_SubSystem2620_SubSystem2624_SubSystem2644_SubSystem2663_single1_1"
  single2/1 -> RO1/2  "mdl5_SubSystem2611_SubSystem2612_SubSystem2620_SubSystem2624_SubSystem2644_SubSystem2663_single2_1"

== system mdl5/SubSystem2611/SubSystem2612/SubSystem2620/SubSystem2624/SubSystem2644/SubSystem2664 ==
  note: ***編集禁止***
  In1 : Inport
  In2 : Inport  Port=2
  RO1 : RelationalOperator  Operator===  InputSameDT=on
  single1 : DataTypeConversion  OutDataTypeStr=single  SaturateOnIntegerOverflow=on  RndMeth=Zero
  single2 : DataTypeConversion  OutDataTypeStr=single  SaturateOnIntegerOverflow=on  RndMeth=Zero
  Out1 : Outport
  wires:
  RO1/1 -> Out1/1  "mdl5_SubSystem2611_SubSystem2612_SubSystem2620_SubSystem2624_SubSystem2644_SubSystem2664_RO1_1"
  In2/1 -> single2/1
  In1/1 -> single1/1
  single1/1 -> RO1/1  "mdl5_SubSystem2611_SubSystem2612_SubSystem2620_SubSystem2624_SubSystem2644_SubSystem2664_single1_1"
  single2/1 -> RO1/2  "mdl5_SubSystem2611_SubSystem2612_SubSystem2620_SubSystem2624_SubSystem2644_SubSystem2664_single2_1"

== system mdl5/SubSystem2611/SubSystem2612/SubSystem2665/SubSystem2666/SubSystem2670/SubSystem2671 ==
  note: ***編集禁止***
  element : Inport
  Inside_DSR : DataStoreRead  DataStoreName=DSM97
  Selector : Selector  IndexOptions=Index vector (port)  Indices=[1 3]
  Output : Outport
  wires:
  Inside_DSR/1 -> Selector/1  "mdl5_SubSystem2611_SubSystem2612_SubSystem2665_SubSystem2666_SubSystem2670_SubSystem2671_Inside_DSR_1"
  element/1 -> Selector/2
  Selector/1 -> Output/1  "mdl5_SubSystem2611_SubSystem2612_SubSystem2665_SubSystem2666_SubSystem2670_SubSystem2671_Selector_1"

== system mdl5/SubSystem2611/SubSystem2612/SubSystem2665/SubSystem2666/SubSystem2670/SubSystem2672 ==
  note: ***編集禁止***
  element : Inport
  Inside_DSR : DataStoreRead  DataStoreName=DSM318
  Selector : Selector  IndexOptions=Index vector (port)  Indices=[1 3]
  Output : Outport
  wires:
  Selector/1 -> Output/1  "mdl5_SubSystem2611_SubSystem2612_SubSystem2665_SubSystem2666_SubSystem2670_SubSystem2672_Selector_1"
  element/1 -> Selector/2
  Inside_DSR/1 -> Selector/1  "mdl5_SubSystem2611_SubSystem2612_SubSystem2665_SubSystem2666_SubSystem2670_SubSystem2672_Inside_DSR_1"

== system mdl5/SubSystem2611/SubSystem2612/SubSystem2665/SubSystem2666/SubSystem2670/SubSystem2673 ==
  note: ***編集禁止***
  element : Inport
  Inside_DSR : DataStoreRead  DataStoreName=DSM36
  Selector : Selector  IndexOptions=Index vector (port)  Indices=[1 3]
  Output : Outport
  wires:
  Inside_DSR/1 -> Selector/1  "mdl5_SubSystem2611_SubSystem2612_SubSystem2665_SubSystem2666_SubSystem2670_SubSystem2673_Inside_DSR_1"
  element/1 -> Selector/2
  Selector/1 -> Output/1  "mdl5_SubSystem2611_SubSystem2612_SubSystem2665_SubSystem2666_SubSystem2670_SubSystem2673_Selector_1"

== system mdl5/SubSystem2611/SubSystem2612/SubSystem2665/SubSystem2666/SubSystem2670/SubSystem2674 ==
  note: ***編集禁止***
  input : Inport
  element : Inport  Port=2
  Assignment : Assignment  IndexOptions=Index vector (port)  OutputSizes=[1 1]
  Inside_DSR : DataStoreRead  DataStoreName=DSM321
  Inside_DSW : DataStoreWrite  DataStoreName=DSM321
  wires:
  element/1 -> Assignment/3
  input/1 -> Assignment/2
  Inside_DSR/1 -> Assignment/1  "mdl5_SubSystem2611_SubSystem2612_SubSystem2665_SubSystem2666_SubSystem2670_SubSystem2674_Inside_DSR_1"
  Assignment/1 -> Inside_DSW/1  "mdl5_SubSystem2611_SubSystem2612_SubSystem2665_SubSystem2666_SubSystem2670_SubSystem2674_Assignment_1"

== system mdl5/SubSystem2611/SubSystem2612/SubSystem2665/SubSystem2666/SubSystem2670/SubSystem2675 ==
  note: ***編集禁止***
  In1 : Inport
  In2 : Inport  Port=2
  RO1 : RelationalOperator  Operator===  InputSameDT=on
  single1 : DataTypeConversion  OutDataTypeStr=single  SaturateOnIntegerOverflow=on  RndMeth=Zero
  single2 : DataTypeConversion  OutDataTypeStr=single  SaturateOnIntegerOverflow=on  RndMeth=Zero
  Out1 : Outport
  wires:
  single2/1 -> RO1/2  "mdl5_SubSystem2611_SubSystem2612_SubSystem2665_SubSystem2666_SubSystem2670_SubSystem2675_single2_1"
  single1/1 -> RO1/1  "mdl5_SubSystem2611_SubSystem2612_SubSystem2665_SubSystem2666_SubSystem2670_SubSystem2675_single1_1"
  In1/1 -> single1/1
  In2/1 -> single2/1
  RO1/1 -> Out1/1  "mdl5_SubSystem2611_SubSystem2612_SubSystem2665_SubSystem2666_SubSystem2670_SubSystem2675_RO1_1"

== system mdl5/SubSystem2611/SubSystem2612/SubSystem2665/SubSystem2666/SubSystem2676/SubSystem2677 ==
  note: ***編集禁止***
  element : Inport
  Inside_DSR : DataStoreRead  DataStoreName=DSM334
  Selector : Selector  IndexOptions=Index vector (port)  Indices=[1 3]
  Output : Outport
  wires:
  Inside_DSR/1 -> Selector/1  "mdl5_SubSystem2611_SubSystem2612_SubSystem2665_SubSystem2666_SubSystem2676_SubSystem2677_Inside_DSR_1"
  element/1 -> Selector/2
  Selector/1 -> Output/1  "mdl5_SubSystem2611_SubSystem2612_SubSystem2665_SubSystem2666_SubSystem2676_SubSystem2677_Selector_1"

== system mdl5/SubSystem2611/SubSystem2612/SubSystem2665/SubSystem2666/SubSystem2676/SubSystem2678 ==
  note: ***編集禁止***
  element : Inport
  Inside_DSR : DataStoreRead  DataStoreName=DSM335
  Selector : Selector  IndexOptions=Index vector (port)  Indices=[1 3]
  Output : Outport
  wires:
  Selector/1 -> Output/1  "mdl5_SubSystem2611_SubSystem2612_SubSystem2665_SubSystem2666_SubSystem2676_SubSystem2678_Selector_1"
  element/1 -> Selector/2
  Inside_DSR/1 -> Selector/1  "mdl5_SubSystem2611_SubSystem2612_SubSystem2665_SubSystem2666_SubSystem2676_SubSystem2678_Inside_DSR_1"

== system mdl5/SubSystem2611/SubSystem2612/SubSystem2665/SubSystem2666/SubSystem2676/SubSystem2679 ==
  note: ***編集禁止***
  element : Inport
  Inside_DSR : DataStoreRead  DataStoreName=DSM336
  Selector : Selector  IndexOptions=Index vector (port)  Indices=[1 3]
  Output : Outport
  wires:
  Inside_DSR/1 -> Selector/1  "mdl5_SubSystem2611_SubSystem2612_SubSystem2665_SubSystem2666_SubSystem2676_SubSystem2679_Inside_DSR_1"
  element/1 -> Selector/2
  Selector/1 -> Output/1  "mdl5_SubSystem2611_SubSystem2612_SubSystem2665_SubSystem2666_SubSystem2676_SubSystem2679_Selector_1"

== system mdl5/SubSystem2611/SubSystem2612/SubSystem2665/SubSystem2666/SubSystem2676/SubSystem2680 ==
  note: ***編集禁止***
  element : Inport
  Inside_DSR : DataStoreRead  DataStoreName=DSM337
  Selector : Selector  IndexOptions=Index vector (port)  Indices=[1 3]
  Output : Outport
  wires:
  Selector/1 -> Output/1  "mdl5_SubSystem2611_SubSystem2612_SubSystem2665_SubSystem2666_SubSystem2676_SubSystem2680_Selector_1"
  element/1 -> Selector/2
  Inside_DSR/1 -> Selector/1  "mdl5_SubSystem2611_SubSystem2612_SubSystem2665_SubSystem2666_SubSystem2676_SubSystem2680_Inside_DSR_1"

== system mdl5/SubSystem2611/SubSystem2612/SubSystem2665/SubSystem2666/SubSystem2676/SubSystem2681 ==
  note: ***編集禁止***
  input : Inport
  element : Inport  Port=2
  Assignment : Assignment  IndexOptions=Index vector (port)  OutputSizes=[1 1]
  Inside_DSR : DataStoreRead  DataStoreName=DSM334
  Inside_DSW : DataStoreWrite  DataStoreName=DSM334
  wires:
  Assignment/1 -> Inside_DSW/1  "mdl5_SubSystem2611_SubSystem2612_SubSystem2665_SubSystem2666_SubSystem2676_SubSystem2681_Assignment_1"
  Inside_DSR/1 -> Assignment/1  "mdl5_SubSystem2611_SubSystem2612_SubSystem2665_SubSystem2666_SubSystem2676_SubSystem2681_Inside_DSR_1"
  input/1 -> Assignment/2
  element/1 -> Assignment/3

== system mdl5/SubSystem2611/SubSystem2612/SubSystem2665/SubSystem2666/SubSystem2676/SubSystem2682 ==
  note: ***編集禁止***
  input : Inport
  element : Inport  Port=2
  Assignment : Assignment  IndexOptions=Index vector (port)  OutputSizes=[1 1]
  Inside_DSR : DataStoreRead  DataStoreName=DSM335
  Inside_DSW : DataStoreWrite  DataStoreName=DSM335
  wires:
  element/1 -> Assignment/3
  input/1 -> Assignment/2
  Inside_DSR/1 -> Assignment/1  "mdl5_SubSystem2611_SubSystem2612_SubSystem2665_SubSystem2666_SubSystem2676_SubSystem2682_Inside_DSR_1"
  Assignment/1 -> Inside_DSW/1  "mdl5_SubSystem2611_SubSystem2612_SubSystem2665_SubSystem2666_SubSystem2676_SubSystem2682_Assignment_1"

== system mdl5/SubSystem2611/SubSystem2612/SubSystem2665/SubSystem2666/SubSystem2676/SubSystem2683 ==
  note: ***編集禁止***
  input : Inport
  element : Inport  Port=2
  Assignment : Assignment  IndexOptions=Index vector (port)  OutputSizes=[1 1]
  Inside_DSR : DataStoreRead  DataStoreName=DSM336
  Inside_DSW : DataStoreWrite  DataStoreName=DSM336
  wires:
  Assignment/1 -> Inside_DSW/1  "mdl5_SubSystem2611_SubSystem2612_SubSystem2665_SubSystem2666_SubSystem2676_SubSystem2683_Assignment_1"
  Inside_DSR/1 -> Assignment/1  "mdl5_SubSystem2611_SubSystem2612_SubSystem2665_SubSystem2666_SubSystem2676_SubSystem2683_Inside_DSR_1"
  input/1 -> Assignment/2
  element/1 -> Assignment/3

== system mdl5/SubSystem2611/SubSystem2612/SubSystem2665/SubSystem2666/SubSystem2676/SubSystem2684 ==
  note: ***編集禁止***
  input : Inport
  element : Inport  Port=2
  Assignment : Assignment  IndexOptions=Index vector (port)  OutputSizes=[1 1]
  Inside_DSR : DataStoreRead  DataStoreName=DSM337
  Inside_DSW : DataStoreWrite  DataStoreName=DSM337
  wires:
  element/1 -> Assignment/3
  input/1 -> Assignment/2
  Inside_DSR/1 -> Assignment/1  "mdl5_SubSystem2611_SubSystem2612_SubSystem2665_SubSystem2666_SubSystem2676_SubSystem2684_Inside_DSR_1"
  Assignment/1 -> Inside_DSW/1  "mdl5_SubSystem2611_SubSystem2612_SubSystem2665_SubSystem2666_SubSystem2676_SubSystem2684_Assignment_1"

== system mdl5/SubSystem2611/SubSystem2612/SubSystem2665/SubSystem2666/SubSystem2676/SubSystem2685 ==
  note: ***編集禁止***
  In1 : Inport
  In2 : Inport  Port=2
  RO1 : RelationalOperator  Operator===  InputSameDT=on
  single1 : DataTypeConversion  OutDataTypeStr=single  SaturateOnIntegerOverflow=on  RndMeth=Zero
  single2 : DataTypeConversion  OutDataTypeStr=single  SaturateOnIntegerOverflow=on  RndMeth=Zero
  Out1 : Outport
  wires:
  RO1/1 -> Out1/1  "mdl5_SubSystem2611_SubSystem2612_SubSystem2665_SubSystem2666_SubSystem2676_SubSystem2685_RO1_1"
  In2/1 -> single2/1
  In1/1 -> single1/1
  single1/1 -> RO1/1  "mdl5_SubSystem2611_SubSystem2612_SubSystem2665_SubSystem2666_SubSystem2676_SubSystem2685_single1_1"
  single2/1 -> RO1/2  "mdl5_SubSystem2611_SubSystem2612_SubSystem2665_SubSystem2666_SubSystem2676_SubSystem2685_single2_1"

== system mdl5/SubSystem2611/SubSystem2612/SubSystem2665/SubSystem2666/SubSystem2676/SubSystem2686 ==
  note: ***編集禁止***
  In1 : Inport
  In2 : Inport  Port=2
  RO1 : RelationalOperator  Operator===  InputSameDT=on
  single1 : DataTypeConversion  OutDataTypeStr=single  SaturateOnIntegerOverflow=on  RndMeth=Zero
  single2 : DataTypeConversion  OutDataTypeStr=single  SaturateOnIntegerOverflow=on  RndMeth=Zero
  Out1 : Outport
  wires:
  RO1/1 -> Out1/1  "mdl5_SubSystem2611_SubSystem2612_SubSystem2665_SubSystem2666_SubSystem2676_SubSystem2686_RO1_1"
  In2/1 -> single2/1
  In1/1 -> single1/1
  single1/1 -> RO1/1  "mdl5_SubSystem2611_SubSystem2612_SubSystem2665_SubSystem2666_SubSystem2676_SubSystem2686_single1_1"
  single2/1 -> RO1/2  "mdl5_SubSystem2611_SubSystem2612_SubSystem2665_SubSystem2666_SubSystem2676_SubSystem2686_single2_1"
